simulink model "afe_abc_inv_psm_2mods"  (R2024b)
settings: Solver=ode1be  StartTime=0.0  StopTime=simlength  FixedStep=tc  MaxStep=tc
undefined symbols (not defined in the file): Adrso, afe_pwm_phase_shift_mod1, afe_pwm_phase_shift_mod2, Amplitude_U, Amplitude_V, Amplitude_W, Aresd, b, Bresd, Cresd, Crso, CTRPIFF_CLIP_RELEASE, dead_time_AFE, dead_time_INV, deepNEGeta, deepNEGxi, deepPOSxi, emf_fb_p, emf_fb_p_ccaller_1, emf_fb_p_ccaller_2, emf_p, emf_p_ccaller_1, emf_p_ccaller_2, enable_two_modules, end_time_LVRT, fPWM_AFE, fPWM_INV, g0_161Hz, g0_500Hz, g1_161Hz, g1_500Hz, i_grid_neg_eta_lim, i_grid_neg_eta_red_lim, i_grid_neg_xi_lim, i_grid_neg_xi_red_lim, i_grid_pos_eta_lim, i_grid_pos_eta_red_lim, ibez, id_lim, ieta_neg_ref_lim, ieta_pos_ref_lim, Igrid_phase_normalization_factor, inv_pwm_phase_shift_mod1, inv_pwm_phase_shift_mod2, iq_lim, ixi_pos_ref_lim, Jm, k_frt_ref, kg, ki_afe, ki_i, ki_rc_neg_grid, ki_rc_pos_grid, ki_vs, ki_w, kp_afe, kp_i, kp_rc_neg_grid, kp_rc_pos_grid, kp_vs ... (+59)
libraries: spsSampleandHoldLib x210, fl_lib x202, nesl_utility x126, simulink x22, cstblocks x18, threephase_inductor_lib x4, single_phase_transformer_lib x3, flexshaft_lib x1, pmsm_uvw_with_harmonics_lib x1
(part 6 of 18)

== system afe_abc_inv_psm_2mods/grid/grid_emulator/3ph_Dyg ==
  Electrical Reference1 : fl_lib/Electrical/Electrical Elements/Electrical Reference
  ph1 : single_phase_transformer_lib/single phase transformer  Lm=Lmu2_trafo H  n1=50*sqrt(3)  n2=50  Rd1=0 Ohm  Rd2=Rd2_trafo Ohm  Ld1=0 H  Ld2=Ld2_trafo H  Rfe=Rm2_trafo Ohm  phi_specify=off  phi_priority=None  phi=0 V*s  phi_nominal_specify=off  phi_nominal_value=1  phi_nominal_unit=V*s  i1_specify=off  i1_priority=None  i1=0 A  i1_nominal_specify=off  i1_nominal_value=1  i1_nominal_unit=A  i2_specify=off  i2_priority=None  i2=0 A  i2_nominal_specify=off  i2_nominal_value=1  i2_nominal_unit=A  ife_specify=off  ife_priority=None  ife=0 A  ife_nominal_specify=off  ife_nominal_value=1  ife_nominal_unit=A  u1_specify=off  u1_priority=None  u1=0 V  u1_nominal_specify=off  u1_nominal_value=1  u1_nominal_unit=V  u2_specify=off  u2_priority=None  u2=0 V  u2_nominal_specify=off  u2_nominal_value=1  u2_nominal_unit=V
      settings: InternalSimscapePortConfiguration="{\"Bottom\":[],\"Left\":[{\"id\":\"u1_p\",\"label\":\"u1(+)\",\"type\":\"foundation.electrical.electrical\"},{\"id\":\"u1_n\",\"label\":\"u1(-)\",\"type\":\"foundation.electrical.electrical\"}],\"Right\":[{\"id\":\"u2_p\",\"label\":\"u2(+)\",\"type\":\"foundation.electrical.electrical\"},{\"id\":\"u2_n\",\"label\":\"u2(-)\",\"type\":\"foundation.electrical.electrical\"}],\"Top\":[]}"
  ph2 : single_phase_transformer_lib/single phase transformer  Lm=Lmu2_trafo H  n1=50*sqrt(3)  n2=50  Rd1=0 Ohm  Rd2=Rd2_trafo Ohm  Ld1=0 H  Ld2=Ld2_trafo H  Rfe=Rm2_trafo Ohm  phi_specify=off  phi_priority=None  phi=0 V*s  phi_nominal_specify=off  phi_nominal_value=1  phi_nominal_unit=V*s  i1_specify=off  i1_priority=None  i1=0 A  i1_nominal_specify=off  i1_nominal_value=1  i1_nominal_unit=A  i2_specify=off  i2_priority=None  i2=0 A  i2_nominal_specify=off  i2_nominal_value=1  i2_nominal_unit=A  ife_specify=off  ife_priority=None  ife=0 A  ife_nominal_specify=off  ife_nominal_value=1  ife_nominal_unit=A  u1_specify=off  u1_priority=None  u1=0 V  u1_nominal_specify=off  u1_nominal_value=1  u1_nominal_unit=V  u2_specify=off  u2_priority=None  u2=0 V  u2_nominal_specify=off  u2_nominal_value=1  u2_nominal_unit=V
      settings: InternalSimscapePortConfiguration="{\"Bottom\":[],\"Left\":[{\"id\":\"u1_p\",\"label\":\"u1(+)\",\"type\":\"foundation.electrical.electrical\"},{\"id\":\"u1_n\",\"label\":\"u1(-)\",\"type\":\"foundation.electrical.electrical\"}],\"Right\":[{\"id\":\"u2_p\",\"label\":\"u2(+)\",\"type\":\"foundation.electrical.electrical\"},{\"id\":\"u2_n\",\"label\":\"u2(-)\",\"type\":\"foundation.electrical.electrical\"}],\"Top\":[]}"
  ph3 : single_phase_transformer_lib/single phase transformer  Lm=Lmu2_trafo H  n1=50*sqrt(3)  n2=50  Rd1=0 Ohm  Rd2=Rd2_trafo Ohm  Ld1=0 H  Ld2=Ld2_trafo H  Rfe=Rm2_trafo Ohm  phi_specify=off  phi_priority=None  phi=0 V*s  phi_nominal_specify=off  phi_nominal_value=1  phi_nominal_unit=V*s  i1_specify=off  i1_priority=None  i1=0 A  i1_nominal_specify=off  i1_nominal_value=1  i1_nominal_unit=A  i2_specify=off  i2_priority=None  i2=0 A  i2_nominal_specify=off  i2_nominal_value=1  i2_nominal_unit=A  ife_specify=off  ife_priority=None  ife=0 A  ife_nominal_specify=off  ife_nominal_value=1  ife_nominal_unit=A  u1_specify=off  u1_priority=None  u1=0 V  u1_nominal_specify=off  u1_nominal_value=1  u1_nominal_unit=V  u2_specify=off  u2_priority=None  u2=0 V  u2_nominal_specify=off  u2_nominal_value=1  u2_nominal_unit=V
      settings: InternalSimscapePortConfiguration="{\"Bottom\":[],\"Left\":[{\"id\":\"u1_p\",\"label\":\"u1(+)\",\"type\":\"foundation.electrical.electrical\"},{\"id\":\"u1_n\",\"label\":\"u1(-)\",\"type\":\"foundation.electrical.electrical\"}],\"Right\":[{\"id\":\"u2_p\",\"label\":\"u2(+)\",\"type\":\"foundation.electrical.electrical\"},{\"id\":\"u2_n\",\"label\":\"u2(-)\",\"type\":\"foundation.electrical.electrical\"}],\"Top\":[]}"
  ua : PMIOPort  Side=Right
  ub : PMIOPort  Port=2  Side=Right
  uc : PMIOPort  Port=3  Side=Right
  Ua : PMIOPort  Port=4  Side=Left
  Ub : PMIOPort  Port=5  Side=Left
  Uc : PMIOPort  Port=6  Side=Left
  connections:
  Electrical Reference1/LConn1 -- ph3/RConn2 -- ph2/RConn2 -- ph1/RConn2
  ph3/RConn1 -- uc/RConn1
  ph1/LConn1 -- ph3/LConn2 -- Ua/RConn1
  ph1/RConn1 -- ua/RConn1
  ph2/RConn1 -- ub/RConn1
  ph1/LConn2 -- ph2/LConn1 -- Ub/RConn1
  Uc/RConn1 -- ph3/LConn1 -- ph2/LConn2

== system afe_abc_inv_psm_2mods/grid/grid_emulator/grid_emulator ==
  phase_gen : Subsystem
  voltage_reference : Subsystem
  voltage_source : Subsystem
  Vma : Outport
  Vmb : Outport  Port=2
  Vmc : Outport  Port=3
  wires:
  phase_gen/1(grid_emu_phase) -> voltage_reference/1(grid_emu_phase)  "grid_emu_phase"
  voltage_source/2(vn_xi) -> voltage_reference/3(Vxi_n)
  voltage_source/1(vp_xi) -> voltage_reference/2(Vxi_p)
  voltage_source/3(vn_eta) -> voltage_reference/4(Veta_n)
  voltage_reference/3(V3_ref) -> Vmc/1
  voltage_reference/1(V1_ref) -> Vma/1
  voltage_reference/2(V2_ref) -> Vmb/1

== system afe_abc_inv_psm_2mods/grid/grid_emulator/threephase_vi_measures ==
  Bus Creator : BusCreator  Inputs=6
  Current Sensor : fl_lib/Electrical/Electrical Sensors/Current Sensor
  Current Sensor1 : fl_lib/Electrical/Electrical Sensors/Current Sensor
  Current Sensor2 : fl_lib/Electrical/Electrical Sensors/Current Sensor
  Electrical Reference1 : fl_lib/Electrical/Electrical Elements/Electrical Reference
  Voltage Sensor : fl_lib/Electrical/Electrical Sensors/Voltage Sensor
  Voltage Sensor1 : fl_lib/Electrical/Electrical Sensors/Voltage Sensor
  Voltage Sensor2 : fl_lib/Electrical/Electrical Sensors/Voltage Sensor
  i : Selector  InputPortWidth=6  IndexOptions=Index vector (dialog)  Indices=[4 5 6]  OutputSizes=1
  i_line_abc/u_line_abc : Scope  NumInputPorts=2
  ia_grid : nesl_utility/PS-Simulink Converter  PhysicalDomain=network_engine_domain  SubClassName=ps_output  LeftPortType=input  RightPortType=output  PseudoPeriodic=off  Frequencies=[]  VectorFormat=1-D array  Unit=A  AffineConversion=off
  ib_grid : nesl_utility/PS-Simulink Converter  PhysicalDomain=network_engine_domain  SubClassName=ps_output  LeftPortType=input  RightPortType=output  PseudoPeriodic=off  Frequencies=[]  VectorFormat=1-D array  Unit=A  AffineConversion=off
  ic_grid : nesl_utility/PS-Simulink Converter  PhysicalDomain=network_engine_domain  SubClassName=ps_output  LeftPortType=input  RightPortType=output  PseudoPeriodic=off  Frequencies=[]  VectorFormat=1-D array  Unit=A  AffineConversion=off
  u : Selector  InputPortWidth=6  IndexOptions=Index vector (dialog)  Indices=[1 2 3]  OutputSizes=1
  ua_grid : nesl_utility/PS-Simulink Converter  PhysicalDomain=network_engine_domain  SubClassName=ps_output  LeftPortType=input  RightPortType=output  PseudoPeriodic=off  Frequencies=[]  VectorFormat=1-D array  Unit=V  AffineConversion=off
  ub_grid : nesl_utility/PS-Simulink Converter  PhysicalDomain=network_engine_domain  SubClassName=ps_output  LeftPortType=input  RightPortType=output  PseudoPeriodic=off  Frequencies=[]  VectorFormat=1-D array  Unit=V  AffineConversion=off
  uc_grid : nesl_utility/PS-Simulink Converter  PhysicalDomain=network_engine_domain  SubClassName=ps_output  LeftPortType=input  RightPortType=output  PseudoPeriodic=off  Frequencies=[]  VectorFormat=1-D array  Unit=V  AffineConversion=off
  Ua : PMIOPort  Side=Left
  ua : PMIOPort  Port=2  Side=Right
  Ub : PMIOPort  Port=3  Side=Left
  ub : PMIOPort  Port=4  Side=Right
  Uc : PMIOPort  Port=5  Side=Left
  uc : PMIOPort  Port=6  Side=Right
  wires:
  Bus Creator/1 -> i/1, u/1  "vi_data"
  ib_grid/1 -> Bus Creator/5  "ib"
  ia_grid/1 -> Bus Creator/4  "ia"
  ic_grid/1 -> Bus Creator/6  "ic"
  ua_grid/1 -> Bus Creator/1  "ua"
  ub_grid/1 -> Bus Creator/2  "ub"
  uc_grid/1 -> Bus Creator/3  "uc"
  i/1 -> i_line_abc/u_line_abc/1
  u/1 -> i_line_abc/u_line_abc/2
  connections:
  Current Sensor1/LConn1 -- Ub/RConn1 -- Voltage Sensor1/LConn1
  Electrical Reference1/LConn1 -- Voltage Sensor/RConn2 -- Voltage Sensor2/RConn2 -- Voltage Sensor1/RConn2
  Voltage Sensor/RConn1 -- ua_grid/LConn1
  Current Sensor/RConn2 -- ua/RConn1
  Voltage Sensor1/RConn1 -- ub_grid/LConn1
  Voltage Sensor2/LConn1 -- Current Sensor2/LConn1 -- Uc/RConn1
  Current Sensor/LConn1 -- Ua/RConn1 -- Voltage Sensor/LConn1
  Current Sensor1/RConn2 -- ub/RConn1
  Voltage Sensor2/RConn1 -- uc_grid/LConn1
  ib_grid/LConn1 -- Current Sensor1/RConn1
  ia_grid/LConn1 -- Current Sensor/RConn1
  ic_grid/LConn1 -- Current Sensor2/RConn1
  Current Sensor2/RConn2 -- uc/RConn1

== system afe_abc_inv_psm_2mods/grid/instantaneus_power/abc2alphabeta ==
  a : Inport
  b : Inport  Port=2
  c : Inport  Port=3
  Gain1 : Gain  Gain=-1/2
  Gain11 : Gain  Gain=-1/2
  Gain2 : Gain  Gain=0
  Gain3 : Gain  Gain=sqrt(3)/2
  Gain4 : Gain  Gain=-sqrt(3)/2
  Gain8 : Gain  Gain=2/3
  Gain9 : Gain  Gain=2/3
  Sum : Sum  Inputs=+++
  Sum1 : Sum  Inputs=+++
  "alpha " : Outport  VectorParamsAs1DForOutWhenUnconnected=off
  "beta " : Outport  Port=2  VectorParamsAs1DForOutWhenUnconnected=off
  wires:
  Gain3/1 -> Sum1/2
  Gain2/1 -> Sum1/1
  Gain11/1 -> Sum/2
  Gain4/1 -> Sum1/3
  Sum1/1 -> Gain9/1
  Gain8/1 -> "alpha "/1
  Sum/1 -> Gain8/1
  c/1 -> Gain4/1, Gain1/1
  Gain9/1 -> "beta "/1
  b/1 -> Gain3/1, Gain11/1
  Gain1/1 -> Sum/3
  a/1 -> Gain2/1, Sum/1

== system afe_abc_inv_psm_2mods/grid/instantaneus_power/abc2alphabeta  ==
  a : Inport
  b : Inport  Port=2
  c : Inport  Port=3
  Gain1 : Gain  Gain=-1/2
  Gain11 : Gain  Gain=-1/2
  Gain2 : Gain  Gain=0
  Gain3 : Gain  Gain=sqrt(3)/2
  Gain4 : Gain  Gain=-sqrt(3)/2
  Gain8 : Gain  Gain=2/3
  Gain9 : Gain  Gain=2/3
  Sum : Sum  Inputs=+++
  Sum1 : Sum  Inputs=+++
  "alpha " : Outport  VectorParamsAs1DForOutWhenUnconnected=off
  "beta " : Outport  Port=2  VectorParamsAs1DForOutWhenUnconnected=off
  wires:
  a/1 -> Sum/1, Gain2/1
  Gain2/1 -> Sum1/1
  Gain9/1 -> "beta "/1
  Gain11/1 -> Sum/2
  c/1 -> Gain1/1, Gain4/1
  Sum/1 -> Gain8/1
  Sum1/1 -> Gain9/1
  Gain1/1 -> Sum/3
  Gain3/1 -> Sum1/2
  Gain4/1 -> Sum1/3
  Gain8/1 -> "alpha "/1
  b/1 -> Gain11/1, Gain3/1

== system afe_abc_inv_psm_2mods/grid/instantaneus_power/moving_avarage ==
  In : Inport
  Gain1 : Gain  Gain=omega_grid_emulator_nom/2/pi  SaturateOnIntegerOverflow=on  OutDataTypeStr=Inherit: Same as input  ParamDataTypeStr=Inherit: Same as input
  Sum4 : Sum  SaturateOnIntegerOverflow=on
  Sum8 : Sum  Inputs=+-  InputSameDT=on  SaturateOnIntegerOverflow=on  OutDataTypeStr=Inherit: Same as first input
  Transport Delay : TransportDelay  DelayTime=2*pi/omega_grid_emulator_nom  BufferSize=2048*4  PadeOrder=2
  Unit Delay2 : UnitDelay  SampleTime=ts_afe  HasFrameUpgradeWarning=on
  kp2 : Gain  Gain=ts_afe  SaturateOnIntegerOverflow=on  OutDataTypeStr=Inherit: Same as input  ParamDataTypeStr=Inherit: Same as input
  Mean : Outport  VectorParamsAs1DForOutWhenUnconnected=off
  wires:
  Transport Delay/1 -> Sum8/2
  Sum4/1 -> Sum8/1, Transport Delay/1, Unit Delay2/1
  Sum8/1 -> Gain1/1
  In/1 -> kp2/1
  Unit Delay2/1 -> Sum4/2
  kp2/1 -> Sum4/1
  Gain1/1 -> Mean/1

== system afe_abc_inv_psm_2mods/grid/instantaneus_power/moving_avarage1 ==
  In : Inport
  Gain1 : Gain  Gain=omega_grid_emulator_nom/2/pi  SaturateOnIntegerOverflow=on  OutDataTypeStr=Inherit: Same as input  ParamDataTypeStr=Inherit: Same as input
  Sum4 : Sum  SaturateOnIntegerOverflow=on
  Sum8 : Sum  Inputs=+-  InputSameDT=on  SaturateOnIntegerOverflow=on  OutDataTypeStr=Inherit: Same as first input
  Transport Delay : TransportDelay  DelayTime=2*pi/omega_grid_emulator_nom  BufferSize=2048*4  PadeOrder=2
  Unit Delay2 : UnitDelay  SampleTime=ts_afe  HasFrameUpgradeWarning=on
  kp2 : Gain  Gain=ts_afe  SaturateOnIntegerOverflow=on  OutDataTypeStr=Inherit: Same as input  ParamDataTypeStr=Inherit: Same as input
  Mean : Outport  VectorParamsAs1DForOutWhenUnconnected=off
  wires:
  Gain1/1 -> Mean/1
  kp2/1 -> Sum4/1
  Unit Delay2/1 -> Sum4/2
  In/1 -> kp2/1
  Sum8/1 -> Gain1/1
  Sum4/1 -> Unit Delay2/1, Transport Delay/1, Sum8/1
  Transport Delay/1 -> Sum8/2

== system afe_abc_inv_psm_2mods/grid/instantaneus_power/rms ==
  In1 : Inport
  Gain : Gain  Gain=n10-1
  Gain1 : Gain  Gain=1/n10
  Math Function : Math  Operator=magnitude^2  SignedPower=on
  Sqrt : Sqrt
  Sum : Sum  Inputs=|++
  Unit Delay : UnitDelay  SampleTime=ts_afe  HasFrameUpgradeWarning=on
  Out1 : Outport  VectorParamsAs1DForOutWhenUnconnected=off
  wires:
  In1/1 -> Math Function/1
  Sum/1 -> Gain1/1
  Gain1/1 -> Sqrt/1, Unit Delay/1
  Unit Delay/1 -> Gain/1
  Math Function/1 -> Sum/1
  Sqrt/1 -> Out1/1
  Gain/1 -> Sum/2

== system afe_abc_inv_psm_2mods/grid/instantaneus_power/rms1 ==
  In1 : Inport
  Gain : Gain  Gain=n10-1
  Gain1 : Gain  Gain=1/n10
  Math Function : Math  Operator=magnitude^2  SignedPower=on
  Sqrt : Sqrt
  Sum : Sum  Inputs=|++
  Unit Delay : UnitDelay  SampleTime=ts_afe  HasFrameUpgradeWarning=on
  Out1 : Outport  VectorParamsAs1DForOutWhenUnconnected=off
  wires:
  Gain/1 -> Sum/2
  Sqrt/1 -> Out1/1
  Math Function/1 -> Sum/1
  Unit Delay/1 -> Gain/1
  Gain1/1 -> Unit Delay/1, Sqrt/1
  Sum/1 -> Gain1/1
  In1/1 -> Math Function/1

== system afe_abc_inv_psm_2mods/grid/instantaneus_power/rms2 ==
  In1 : Inport
  Gain : Gain  Gain=n10-1
  Gain1 : Gain  Gain=1/n10
  Math Function : Math  Operator=magnitude^2  SignedPower=on
  Sqrt : Sqrt
  Sum : Sum  Inputs=|++
  Unit Delay : UnitDelay  SampleTime=ts_afe  HasFrameUpgradeWarning=on
  Out1 : Outport  VectorParamsAs1DForOutWhenUnconnected=off
  wires:
  In1/1 -> Math Function/1
  Sum/1 -> Gain1/1
  Gain1/1 -> Sqrt/1, Unit Delay/1
  Unit Delay/1 -> Gain/1
  Math Function/1 -> Sum/1
  Sqrt/1 -> Out1/1
  Gain/1 -> Sum/2

== system afe_abc_inv_psm_2mods/grid/instantaneus_power/rms3 ==
  In1 : Inport
  Gain : Gain  Gain=n10-1
  Gain1 : Gain  Gain=1/n10
  Math Function : Math  Operator=magnitude^2  SignedPower=on
  Sqrt : Sqrt
  Sum : Sum  Inputs=|++
  Unit Delay : UnitDelay  SampleTime=ts_afe  HasFrameUpgradeWarning=on
  Out1 : Outport  VectorParamsAs1DForOutWhenUnconnected=off
  wires:
  Gain/1 -> Sum/2
  Sqrt/1 -> Out1/1
  Math Function/1 -> Sum/1
  Unit Delay/1 -> Gain/1
  Gain1/1 -> Unit Delay/1, Sqrt/1
  Sum/1 -> Gain1/1
  In1/1 -> Math Function/1

== system afe_abc_inv_psm_2mods/grid/instantaneus_power/rms4 ==
  In1 : Inport
  Gain : Gain  Gain=n10-1
  Gain1 : Gain  Gain=1/n10
  Math Function : Math  Operator=magnitude^2  SignedPower=on
  Sqrt : Sqrt
  Sum : Sum  Inputs=|++
  Unit Delay : UnitDelay  SampleTime=ts_afe  HasFrameUpgradeWarning=on
  Out1 : Outport  VectorParamsAs1DForOutWhenUnconnected=off
  wires:
  In1/1 -> Math Function/1
  Sum/1 -> Gain1/1
  Gain1/1 -> Sqrt/1, Unit Delay/1
  Unit Delay/1 -> Gain/1
  Math Function/1 -> Sum/1
  Sqrt/1 -> Out1/1
  Gain/1 -> Sum/2

== system afe_abc_inv_psm_2mods/grid/instantaneus_power/rms5 ==
  In1 : Inport
  Gain : Gain  Gain=n10-1
  Gain1 : Gain  Gain=1/n10
  Math Function : Math  Operator=magnitude^2  SignedPower=on
  Sqrt : Sqrt
  Sum : Sum  Inputs=|++
  Unit Delay : UnitDelay  SampleTime=ts_afe  HasFrameUpgradeWarning=on
  Out1 : Outport  VectorParamsAs1DForOutWhenUnconnected=off
  wires:
  Gain/1 -> Sum/2
  Sqrt/1 -> Out1/1
  Math Function/1 -> Sum/1
  Unit Delay/1 -> Gain/1
  Gain1/1 -> Unit Delay/1, Sqrt/1
  Sum/1 -> Gain1/1
  In1/1 -> Math Function/1

== system afe_abc_inv_psm_2mods/grid/sequences/moving_avarage ==
  In : Inport
  Gain1 : Gain  Gain=omega_grid_emulator_nom/2/pi  SaturateOnIntegerOverflow=on  OutDataTypeStr=Inherit: Same as input  ParamDataTypeStr=Inherit: Same as input
  Sum4 : Sum  SaturateOnIntegerOverflow=on
  Sum8 : Sum  Inputs=+-  InputSameDT=on  SaturateOnIntegerOverflow=on  OutDataTypeStr=Inherit: Same as first input
  Transport Delay : TransportDelay  DelayTime=2*pi/omega_grid_emulator_nom  BufferSize=2048*4  PadeOrder=2
  Unit Delay2 : UnitDelay  SampleTime=ts_afe  HasFrameUpgradeWarning=on
  kp2 : Gain  Gain=ts_afe  SaturateOnIntegerOverflow=on  OutDataTypeStr=Inherit: Same as input  ParamDataTypeStr=Inherit: Same as input
  Mean : Outport  VectorParamsAs1DForOutWhenUnconnected=off
  wires:
  Transport Delay/1 -> Sum8/2
  Sum4/1 -> Sum8/1, Transport Delay/1, Unit Delay2/1
  Sum8/1 -> Gain1/1
  In/1 -> kp2/1
  Unit Delay2/1 -> Sum4/2
  kp2/1 -> Sum4/1
  Gain1/1 -> Mean/1

== system afe_abc_inv_psm_2mods/grid/sequences/moving_avarage1 ==
  In : Inport
  Gain1 : Gain  Gain=omega_grid_emulator_nom/2/pi  SaturateOnIntegerOverflow=on  OutDataTypeStr=Inherit: Same as input  ParamDataTypeStr=Inherit: Same as input
  Sum4 : Sum  SaturateOnIntegerOverflow=on
  Sum8 : Sum  Inputs=+-  InputSameDT=on  SaturateOnIntegerOverflow=on  OutDataTypeStr=Inherit: Same as first input
  Transport Delay : TransportDelay  DelayTime=2*pi/omega_grid_emulator_nom  BufferSize=2048*4  PadeOrder=2
  Unit Delay2 : UnitDelay  SampleTime=ts_afe  HasFrameUpgradeWarning=on
  kp2 : Gain  Gain=ts_afe  SaturateOnIntegerOverflow=on  OutDataTypeStr=Inherit: Same as input  ParamDataTypeStr=Inherit: Same as input
  Mean : Outport  VectorParamsAs1DForOutWhenUnconnected=off
  wires:
  Gain1/1 -> Mean/1
  kp2/1 -> Sum4/1
  Unit Delay2/1 -> Sum4/2
  In/1 -> kp2/1
  Sum8/1 -> Gain1/1
  Sum4/1 -> Unit Delay2/1, Transport Delay/1, Sum8/1
  Transport Delay/1 -> Sum8/2

== system afe_abc_inv_psm_2mods/grid/sequences/moving_avarage10 ==
  In : Inport
  Gain1 : Gain  Gain=omega_grid_emulator_nom/2/pi  SaturateOnIntegerOverflow=on  OutDataTypeStr=Inherit: Same as input  ParamDataTypeStr=Inherit: Same as input
  Sum4 : Sum  SaturateOnIntegerOverflow=on
  Sum8 : Sum  Inputs=+-  InputSameDT=on  SaturateOnIntegerOverflow=on  OutDataTypeStr=Inherit: Same as first input
  Transport Delay : TransportDelay  DelayTime=2*pi/omega_grid_emulator_nom  BufferSize=2048*4  PadeOrder=2
  Unit Delay2 : UnitDelay  SampleTime=ts_afe  HasFrameUpgradeWarning=on
  kp2 : Gain  Gain=ts_afe  SaturateOnIntegerOverflow=on  OutDataTypeStr=Inherit: Same as input  ParamDataTypeStr=Inherit: Same as input
  Mean : Outport  VectorParamsAs1DForOutWhenUnconnected=off
  wires:
  Transport Delay/1 -> Sum8/2
  Sum4/1 -> Sum8/1, Transport Delay/1, Unit Delay2/1
  Sum8/1 -> Gain1/1
  In/1 -> kp2/1
  Unit Delay2/1 -> Sum4/2
  kp2/1 -> Sum4/1
  Gain1/1 -> Mean/1

== system afe_abc_inv_psm_2mods/grid/sequences/moving_avarage11 ==
  In : Inport
  Gain1 : Gain  Gain=omega_grid_emulator_nom/2/pi  SaturateOnIntegerOverflow=on  OutDataTypeStr=Inherit: Same as input  ParamDataTypeStr=Inherit: Same as input
  Sum4 : Sum  SaturateOnIntegerOverflow=on
  Sum8 : Sum  Inputs=+-  InputSameDT=on  SaturateOnIntegerOverflow=on  OutDataTypeStr=Inherit: Same as first input
  Transport Delay : TransportDelay  DelayTime=2*pi/omega_grid_emulator_nom  BufferSize=2048*4  PadeOrder=2
  Unit Delay2 : UnitDelay  SampleTime=ts_afe  HasFrameUpgradeWarning=on
  kp2 : Gain  Gain=ts_afe  SaturateOnIntegerOverflow=on  OutDataTypeStr=Inherit: Same as input  ParamDataTypeStr=Inherit: Same as input
  Mean : Outport  VectorParamsAs1DForOutWhenUnconnected=off
  wires:
  Gain1/1 -> Mean/1
  kp2/1 -> Sum4/1
  Unit Delay2/1 -> Sum4/2
  In/1 -> kp2/1
  Sum8/1 -> Gain1/1
  Sum4/1 -> Unit Delay2/1, Transport Delay/1, Sum8/1
  Transport Delay/1 -> Sum8/2

== system afe_abc_inv_psm_2mods/grid/sequences/moving_avarage2 ==
  In : Inport
  Gain1 : Gain  Gain=omega_grid_emulator_nom/2/pi  SaturateOnIntegerOverflow=on  OutDataTypeStr=Inherit: Same as input  ParamDataTypeStr=Inherit: Same as input
  Sum4 : Sum  SaturateOnIntegerOverflow=on
  Sum8 : Sum  Inputs=+-  InputSameDT=on  SaturateOnIntegerOverflow=on  OutDataTypeStr=Inherit: Same as first input
  Transport Delay : TransportDelay  DelayTime=2*pi/omega_grid_emulator_nom  BufferSize=2048*4  PadeOrder=2
  Unit Delay2 : UnitDelay  SampleTime=ts_afe  HasFrameUpgradeWarning=on
  kp2 : Gain  Gain=ts_afe  SaturateOnIntegerOverflow=on  OutDataTypeStr=Inherit: Same as input  ParamDataTypeStr=Inherit: Same as input
  Mean : Outport  VectorParamsAs1DForOutWhenUnconnected=off
  wires:
  Transport Delay/1 -> Sum8/2
  Sum4/1 -> Sum8/1, Transport Delay/1, Unit Delay2/1
  Sum8/1 -> Gain1/1
  In/1 -> kp2/1
  Unit Delay2/1 -> Sum4/2
  kp2/1 -> Sum4/1
  Gain1/1 -> Mean/1

== system afe_abc_inv_psm_2mods/grid/sequences/moving_avarage3 ==
  In : Inport
  Gain1 : Gain  Gain=omega_grid_emulator_nom/2/pi  SaturateOnIntegerOverflow=on  OutDataTypeStr=Inherit: Same as input  ParamDataTypeStr=Inherit: Same as input
  Sum4 : Sum  SaturateOnIntegerOverflow=on
  Sum8 : Sum  Inputs=+-  InputSameDT=on  SaturateOnIntegerOverflow=on  OutDataTypeStr=Inherit: Same as first input
  Transport Delay : TransportDelay  DelayTime=2*pi/omega_grid_emulator_nom  BufferSize=2048*4  PadeOrder=2
  Unit Delay2 : UnitDelay  SampleTime=ts_afe  HasFrameUpgradeWarning=on
  kp2 : Gain  Gain=ts_afe  SaturateOnIntegerOverflow=on  OutDataTypeStr=Inherit: Same as input  ParamDataTypeStr=Inherit: Same as input
  Mean : Outport  VectorParamsAs1DForOutWhenUnconnected=off
  wires:
  Gain1/1 -> Mean/1
  kp2/1 -> Sum4/1
  Unit Delay2/1 -> Sum4/2
  In/1 -> kp2/1
  Sum8/1 -> Gain1/1
  Sum4/1 -> Unit Delay2/1, Transport Delay/1, Sum8/1
  Transport Delay/1 -> Sum8/2

== system afe_abc_inv_psm_2mods/grid/sequences/moving_avarage4 ==
  In : Inport
  Gain1 : Gain  Gain=omega_grid_emulator_nom/2/pi  SaturateOnIntegerOverflow=on  OutDataTypeStr=Inherit: Same as input  ParamDataTypeStr=Inherit: Same as input
  Sum4 : Sum  SaturateOnIntegerOverflow=on
  Sum8 : Sum  Inputs=+-  InputSameDT=on  SaturateOnIntegerOverflow=on  OutDataTypeStr=Inherit: Same as first input
  Transport Delay : TransportDelay  DelayTime=2*pi/omega_grid_emulator_nom  BufferSize=2048*4  PadeOrder=2
  Unit Delay2 : UnitDelay  SampleTime=ts_afe  HasFrameUpgradeWarning=on
  kp2 : Gain  Gain=ts_afe  SaturateOnIntegerOverflow=on  OutDataTypeStr=Inherit: Same as input  ParamDataTypeStr=Inherit: Same as input
  Mean : Outport  VectorParamsAs1DForOutWhenUnconnected=off
  wires:
  Transport Delay/1 -> Sum8/2
  Sum4/1 -> Sum8/1, Transport Delay/1, Unit Delay2/1
  Sum8/1 -> Gain1/1
  In/1 -> kp2/1
  Unit Delay2/1 -> Sum4/2
  kp2/1 -> Sum4/1
  Gain1/1 -> Mean/1

== system afe_abc_inv_psm_2mods/grid/sequences/moving_avarage5 ==
  In : Inport
  Gain1 : Gain  Gain=omega_grid_emulator_nom/2/pi  SaturateOnIntegerOverflow=on  OutDataTypeStr=Inherit: Same as input  ParamDataTypeStr=Inherit: Same as input
  Sum4 : Sum  SaturateOnIntegerOverflow=on
  Sum8 : Sum  Inputs=+-  InputSameDT=on  SaturateOnIntegerOverflow=on  OutDataTypeStr=Inherit: Same as first input
  Transport Delay : TransportDelay  DelayTime=2*pi/omega_grid_emulator_nom  BufferSize=2048*4  PadeOrder=2
  Unit Delay2 : UnitDelay  SampleTime=ts_afe  HasFrameUpgradeWarning=on
  kp2 : Gain  Gain=ts_afe  SaturateOnIntegerOverflow=on  OutDataTypeStr=Inherit: Same as input  ParamDataTypeStr=Inherit: Same as input
  Mean : Outport  VectorParamsAs1DForOutWhenUnconnected=off
  wires:
  Gain1/1 -> Mean/1
  kp2/1 -> Sum4/1
  Unit Delay2/1 -> Sum4/2
  In/1 -> kp2/1
  Sum8/1 -> Gain1/1
  Sum4/1 -> Unit Delay2/1, Transport Delay/1, Sum8/1
  Transport Delay/1 -> Sum8/2

== system afe_abc_inv_psm_2mods/grid/sequences/moving_avarage6 ==
  In : Inport
  Gain1 : Gain  Gain=omega_grid_emulator_nom/2/pi  SaturateOnIntegerOverflow=on  OutDataTypeStr=Inherit: Same as input  ParamDataTypeStr=Inherit: Same as input
  Sum4 : Sum  SaturateOnIntegerOverflow=on
  Sum8 : Sum  Inputs=+-  InputSameDT=on  SaturateOnIntegerOverflow=on  OutDataTypeStr=Inherit: Same as first input
  Transport Delay : TransportDelay  DelayTime=2*pi/omega_grid_emulator_nom  BufferSize=2048*4  PadeOrder=2
  Unit Delay2 : UnitDelay  SampleTime=ts_afe  HasFrameUpgradeWarning=on
  kp2 : Gain  Gain=ts_afe  SaturateOnIntegerOverflow=on  OutDataTypeStr=Inherit: Same as input  ParamDataTypeStr=Inherit: Same as input
  Mean : Outport  VectorParamsAs1DForOutWhenUnconnected=off
  wires:
  Transport Delay/1 -> Sum8/2
  Sum4/1 -> Sum8/1, Transport Delay/1, Unit Delay2/1
  Sum8/1 -> Gain1/1
  In/1 -> kp2/1
  Unit Delay2/1 -> Sum4/2
  kp2/1 -> Sum4/1
  Gain1/1 -> Mean/1

== system afe_abc_inv_psm_2mods/grid/sequences/moving_avarage7 ==
  In : Inport
  Gain1 : Gain  Gain=omega_grid_emulator_nom/2/pi  SaturateOnIntegerOverflow=on  OutDataTypeStr=Inherit: Same as input  ParamDataTypeStr=Inherit: Same as input
  Sum4 : Sum  SaturateOnIntegerOverflow=on
  Sum8 : Sum  Inputs=+-  InputSameDT=on  SaturateOnIntegerOverflow=on  OutDataTypeStr=Inherit: Same as first input
  Transport Delay : TransportDelay  DelayTime=2*pi/omega_grid_emulator_nom  BufferSize=2048*4  PadeOrder=2
  Unit Delay2 : UnitDelay  SampleTime=ts_afe  HasFrameUpgradeWarning=on
  kp2 : Gain  Gain=ts_afe  SaturateOnIntegerOverflow=on  OutDataTypeStr=Inherit: Same as input  ParamDataTypeStr=Inherit: Same as input
  Mean : Outport  VectorParamsAs1DForOutWhenUnconnected=off
  wires:
  Gain1/1 -> Mean/1
  kp2/1 -> Sum4/1
  Unit Delay2/1 -> Sum4/2
  In/1 -> kp2/1
  Sum8/1 -> Gain1/1
  Sum4/1 -> Unit Delay2/1, Transport Delay/1, Sum8/1
  Transport Delay/1 -> Sum8/2

== system afe_abc_inv_psm_2mods/grid/sequences/moving_avarage8 ==
  In : Inport
  Gain1 : Gain  Gain=omega_grid_emulator_nom/2/pi  SaturateOnIntegerOverflow=on  OutDataTypeStr=Inherit: Same as input  ParamDataTypeStr=Inherit: Same as input
  Sum4 : Sum  SaturateOnIntegerOverflow=on
  Sum8 : Sum  Inputs=+-  InputSameDT=on  SaturateOnIntegerOverflow=on  OutDataTypeStr=Inherit: Same as first input
  Transport Delay : TransportDelay  DelayTime=2*pi/omega_grid_emulator_nom  BufferSize=2048*4  PadeOrder=2
  Unit Delay2 : UnitDelay  SampleTime=ts_afe  HasFrameUpgradeWarning=on
  kp2 : Gain  Gain=ts_afe  SaturateOnIntegerOverflow=on  OutDataTypeStr=Inherit: Same as input  ParamDataTypeStr=Inherit: Same as input
  Mean : Outport  VectorParamsAs1DForOutWhenUnconnected=off
  wires:
  Transport Delay/1 -> Sum8/2
  Sum4/1 -> Sum8/1, Transport Delay/1, Unit Delay2/1
  Sum8/1 -> Gain1/1
  In/1 -> kp2/1
  Unit Delay2/1 -> Sum4/2
  kp2/1 -> Sum4/1
  Gain1/1 -> Mean/1

== system afe_abc_inv_psm_2mods/grid/sequences/moving_avarage9 ==
  In : Inport
  Gain1 : Gain  Gain=omega_grid_emulator_nom/2/pi  SaturateOnIntegerOverflow=on  OutDataTypeStr=Inherit: Same as input  ParamDataTypeStr=Inherit: Same as input
  Sum4 : Sum  SaturateOnIntegerOverflow=on
  Sum8 : Sum  Inputs=+-  InputSameDT=on  SaturateOnIntegerOverflow=on  OutDataTypeStr=Inherit: Same as first input
  Transport Delay : TransportDelay  DelayTime=2*pi/omega_grid_emulator_nom  BufferSize=2048*4  PadeOrder=2
  Unit Delay2 : UnitDelay  SampleTime=ts_afe  HasFrameUpgradeWarning=on
  kp2 : Gain  Gain=ts_afe  SaturateOnIntegerOverflow=on  OutDataTypeStr=Inherit: Same as input  ParamDataTypeStr=Inherit: Same as input
  Mean : Outport  VectorParamsAs1DForOutWhenUnconnected=off
  wires:
  Gain1/1 -> Mean/1
  kp2/1 -> Sum4/1
  Unit Delay2/1 -> Sum4/2
  In/1 -> kp2/1
  Sum8/1 -> Gain1/1
  Sum4/1 -> Unit Delay2/1, Transport Delay/1, Sum8/1
  Transport Delay/1 -> Sum8/2

== system afe_abc_inv_psm_2mods/afe_abc_inv_psm_mod1/afe/dclink_measure/R_derating ==
  Step : Step  After=107.4e3/2  SampleTime=0
  Step1 : Step  Time=1.1  After=-107.4e3/2  SampleTime=0
  Sum : Sum  Inputs=|++
  DR : Outport
  wires:
  Step1/1 -> Sum/2
  Step/1 -> Sum/1
  Sum/1 -> DR/1

== system afe_abc_inv_psm_2mods/afe_abc_inv_psm_mod1/afe/dclink_measure/Subsystem1 ==
  In : Inport
  Sample and Hold : spsSampleandHoldLib/Sample and Hold  ic=0  Ts=0
  Out : Outport
  wires:
  Sample and Hold/1 -> Out/1
  [TRGO_afe_module_1] -> Sample and Hold/2
  In/1 -> Sample and Hold/1

== system afe_abc_inv_psm_2mods/afe_abc_inv_psm_mod1/afe/dclink_measure/Subsystem2 ==
  In : Inport
  Sample and Hold : spsSampleandHoldLib/Sample and Hold  ic=0  Ts=0
  Out : Outport
  wires:
  Sample and Hold/1 -> Out/1
  [TRGO_inv_module_1] -> Sample and Hold/2
  In/1 -> Sample and Hold/1

== system afe_abc_inv_psm_2mods/afe_abc_inv_psm_mod1/afe/sv_pwm/Subsystem1 ==
  In : Inport
  Sample and Hold : spsSampleandHoldLib/Sample and Hold  ic=0  Ts=0
  Out : Outport
  wires:
  In/1 -> Sample and Hold/1
  [TRGO_afe_module_1] -> Sample and Hold/2
  Sample and Hold/1 -> Out/1

== system afe_abc_inv_psm_2mods/afe_abc_inv_psm_mod1/afe/sv_pwm/Subsystem2 ==
  In : Inport
  Sample and Hold : spsSampleandHoldLib/Sample and Hold  ic=0  Ts=0
  Out : Outport
  wires:
  Sample and Hold/1 -> Out/1
  [TRGO_afe_module_1] -> Sample and Hold/2
  In/1 -> Sample and Hold/1

== system afe_abc_inv_psm_2mods/afe_abc_inv_psm_mod1/afe/sv_pwm/Subsystem4 ==
  In : Inport
  Sample and Hold : spsSampleandHoldLib/Sample and Hold  ic=0  Ts=0
  Out : Outport
  wires:
  Sample and Hold/1 -> Out/1
  [TRGO_afe_module_1] -> Sample and Hold/2
  In/1 -> Sample and Hold/1

== system afe_abc_inv_psm_2mods/afe_abc_inv_psm_mod1/afe/sv_pwm/Subsystem5 ==
  In : Inport
  Sample and Hold : spsSampleandHoldLib/Sample and Hold  ic=0  Ts=0
  Out : Outport
  wires:
  In/1 -> Sample and Hold/1
  [TRGO_afe_module_1] -> Sample and Hold/2
  Sample and Hold/1 -> Out/1

== system afe_abc_inv_psm_2mods/afe_abc_inv_psm_mod1/afe/sv_pwm/modulator1 ==
  u : Inport
  v : Inport  Port=2
  w : Inport  Port=3
  phase : Inport  Port=4
  Bus Creator3 : BusCreator  Inputs=6
  PWM generator 1 : Subsystem  mask{f=fPWM_AFE, m_up=0.98, m_low=0.02, dead_time=dead_time_AFE, pos_cmd_gate=15, neg_cmd_gate=-10, polarity=1}
      mask prompts: f "Frequency (Hz)"; m_up "Max Input Modulation Value"; m_low "Min Input Modulation Value"; dead_time "Dead Time (s)"; pos_cmd_gate "Positive Gate Voltage (V)"; neg_cmd_gate "Negative Gate Voltage (V)"; polarity "Polarity (pu)"
  PWM generator 2 : Subsystem  mask{f=fPWM_AFE, m_up=0.98, m_low=0.02, dead_time=dead_time_AFE, pos_cmd_gate=15, neg_cmd_gate=-10, polarity=1}
      mask prompts: f "Frequency (Hz)"; m_up "Max Input Modulation Value"; m_low "Min Input Modulation Value"; dead_time "Dead Time (s)"; pos_cmd_gate "Positive Gate Voltage (V)"; neg_cmd_gate "Negative Gate Voltage (V)"; polarity "Polarity (pu)"
  PWM generator 3 : Subsystem  mask{f=fPWM_AFE, m_up=0.98, m_low=0.02, dead_time=dead_time_AFE, pos_cmd_gate=15, neg_cmd_gate=-10, polarity=1}
      mask prompts: f "Frequency (Hz)"; m_up "Max Input Modulation Value"; m_low "Min Input Modulation Value"; dead_time "Dead Time (s)"; pos_cmd_gate "Positive Gate Voltage (V)"; neg_cmd_gate "Negative Gate Voltage (V)"; polarity "Polarity (pu)"
  cmd_gates : Outport
  wires:
  u/1 -> PWM generator 1/1(m_index)
  w/1 -> PWM generator 3/1(m_index)
  v/1 -> PWM generator 2/1(m_index)
  phase/1 -> PWM generator 3/2(phase), PWM generator 2/2(phase), PWM generator 1/2(phase)
  PWM generator 1/2(m2) -> Bus Creator3/2  "pwm_afe_phase_u_bottom"
  PWM generator 3/1(m1) -> Bus Creator3/5  "pwm_afe_phase_w_top"
  PWM generator 2/1(m1) -> Bus Creator3/3  "pwm_afe_phase_v_top"
  PWM generator 2/2(m2) -> Bus Creator3/4  "pwm_afe_phase_v_bottom"
  PWM generator 3/2(m2) -> Bus Creator3/6  "pwm_afe_phase_w_bottom"
  PWM generator 1/1(m1) -> Bus Creator3/1  "pwm_afe_phase_u_top"
  Bus Creator3/1 -> cmd_gates/1

== system afe_abc_inv_psm_2mods/afe_abc_inv_psm_mod1/afe_control/FRT-VDE4110/FRT-Detection ==
  red_dyn_enabled : Inport
  Abs : Abs  SaturateOnIntegerOverflow=off
  Abs1 : Abs  SaturateOnIntegerOverflow=off
  LVRT_detector : MATLAB Function  TreatAsAtomicUnit=on  SystemSampleTime=ts_afe
  Step1 : Step  Time=0.025  Before=1  After=0  SampleTime=ts_afe
  Step3 : Step  Time=settle_time  SampleTime=ts_afe
  dvxi_n/dt : Subsystem
  dvxi_p/dt : Subsystem
  frt_detection_inputs : Scope  NumInputPorts=6
  frt_exceeded : Outport
  frt_state : Outport  Port=2
  red_dyn_active : Outport  Port=3
  frt_active : Outport  Port=4
  pwr_lim_enable : Outport  Port=5
  wires:
  [v_grid_neg_xi_avg_mod1] -> LVRT_detector/2(vxi_n), frt_detection_inputs/2, dvxi_n/dt/1(x)  "v_grid_neg_xi_avg"
  [v_grid_pos_xi_avg_mod1] -> LVRT_detector/1(vxi_p), frt_detection_inputs/1, dvxi_p/dt/1(x)  "v_grid_pos_xi_avg"
  [v_grid_neg_eta_avg_mod1] -> LVRT_detector/3(veta_n), frt_detection_inputs/3  "v_grid_neg_eta_avg"
  Step3/1 -> frt_detection_inputs/6, LVRT_detector/6(enable)  "enable"
  dvxi_p/dt/1(xdot_hat) -> Abs/1
  LVRT_detector/1(pwr_lim_enable) -> pwr_lim_enable/1  "pwr_lim_enable"
  dvxi_n/dt/1(xdot_hat) -> Abs1/1
  Step1/1 -> LVRT_detector/8(reset)
  red_dyn_enabled/1 -> LVRT_detector/7(red_dyn_enabled)
  LVRT_detector/2(frt_exceeded) -> frt_exceeded/1  "lvrt_exceeded"
  LVRT_detector/5(red_dyn_active) -> red_dyn_active/1
  LVRT_detector/4(frt_state) -> frt_state/1
  LVRT_detector/3(frt_active) -> frt_active/1
  Abs/1 -> frt_detection_inputs/4, LVRT_detector/4(vxi_p_dot)  "vxi_pos_dot"
  Abs1/1 -> frt_detection_inputs/5, LVRT_detector/5(vxi_n_dot)  "vxi_neg_dot"

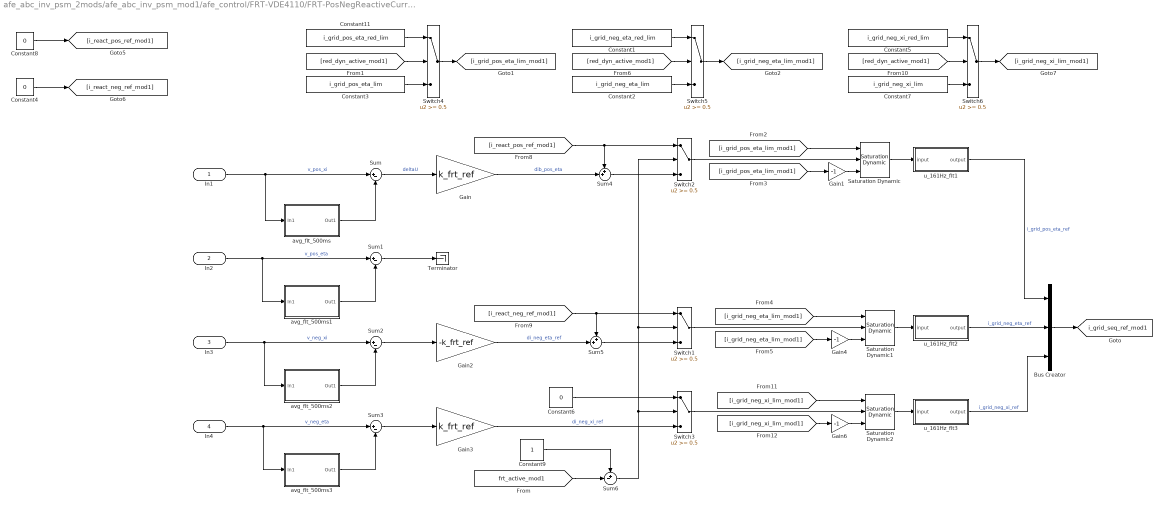
== system afe_abc_inv_psm_2mods/afe_abc_inv_psm_mod1/afe_control/FRT-VDE4110/FRT-PosNegReactiveCurrentReferences ==
  In1 : Inport
  In2 : Inport  Port=2
  In3 : Inport  Port=3
  In4 : Inport  Port=4
  Bus Creator : BusCreator  Inputs=3
  Constant1 : Constant  Value=i_grid_neg_eta_red_lim
  Constant11 : Constant  Value=i_grid_pos_eta_red_lim
  Constant2 : Constant  Value=i_grid_neg_eta_lim
  Constant3 : Constant  Value=i_grid_pos_eta_lim
  Constant4 : Constant  Value=0
  Constant5 : Constant  Value=i_grid_neg_xi_red_lim
  Constant6 : Constant  Value=0
  Constant7 : Constant  Value=i_grid_neg_xi_lim
  Constant8 : Constant  Value=0
  Constant9 : Constant
  Gain : Gain  Gain=k_frt_ref
  Gain1 : Gain  Gain=-1
  Gain2 : Gain  Gain=-k_frt_ref
  Gain3 : Gain  Gain=k_frt_ref
  Gain4 : Gain  Gain=-1
  Gain6 : Gain  Gain=-1
  Saturation Dynamic : simulink/Discontinuities/Saturation Dynamic  OutMin=[]  OutMax=[]  OutDataTypeStr=Inherit: Same as second input  OutDataType=fixdt(1, 16)  OutScaling=2^-10  DoSatur=off
  Saturation Dynamic1 : simulink/Discontinuities/Saturation Dynamic  OutMin=[]  OutMax=[]  OutDataTypeStr=Inherit: Same as second input  OutDataType=fixdt(1, 16)  OutScaling=2^-10  DoSatur=off
  Saturation Dynamic2 : simulink/Discontinuities/Saturation Dynamic  OutMin=[]  OutMax=[]  OutDataTypeStr=Inherit: Same as second input  OutDataType=fixdt(1, 16)  OutScaling=2^-10  DoSatur=off
  Sum{,1..3} (4 alike) : Sum  Inputs=|+-
  Sum4 : Sum  Inputs=++|
  Sum5 : Sum  Inputs=++|
  Sum6 : Sum  Inputs=+-|
  Switch{1..6} (6 alike) : Switch  Threshold=0.5  SaturateOnIntegerOverflow=off  InputSameDT=off
  Terminator : Terminator
  avg_flt_500ms : Subsystem
  avg_flt_500ms1 : Subsystem
  avg_flt_500ms2 : Subsystem
  avg_flt_500ms3 : Subsystem
  u_161Hz_flt1 : Subsystem
  u_161Hz_flt2 : Subsystem
  u_161Hz_flt3 : Subsystem
  tag scope: i_grid_seq_ref_mod1=global
  wires:
  In1/1 -> avg_flt_500ms/1(In1), Sum/1  "v_pos_xi"
  avg_flt_500ms/1(Out1) -> Sum/2
  Sum/1 -> Gain/1  "deltaU"
  Sum1/1 -> Terminator/1
  avg_flt_500ms1/1(Out1) -> Sum1/2
  In2/1 -> avg_flt_500ms1/1(In1), Sum1/1  "v_pos_eta"
  avg_flt_500ms3/1(Out1) -> Sum3/2
  Sum2/1 -> Gain2/1
  In3/1 -> avg_flt_500ms2/1(In1), Sum2/1  "v_neg_xi"
  avg_flt_500ms2/1(Out1) -> Sum2/2
  In4/1 -> avg_flt_500ms3/1(In1), Sum3/1  "v_neg_eta"
  Bus Creator/1 -> [i_grid_seq_ref_mod1]
  Gain/1 -> Sum4/2  "dib_pos_eta"
  [i_react_pos_ref_mod1] -> Switch2/1, Sum4/1
  Sum4/1 -> Switch2/3
  Switch2/1 -> Saturation Dynamic/2
  Saturation Dynamic/1 -> u_161Hz_flt1/1(input)
  Constant6/1 -> Switch3/1
  Gain3/1 -> Switch3/3  "di_neg_xi_ref"
  Sum6/1 -> Switch1/2, Switch2/2, Switch3/2
  Sum3/1 -> Gain3/1
  Gain2/1 -> Sum5/2  "di_neg_eta_ref"
  Sum5/1 -> Switch1/3
  [i_react_neg_ref_mod1] -> Switch1/1, Sum5/1
  Switch4/1 -> [i_grid_pos_eta_lim_mod1]
  [red_dyn_active_mod1] -> Switch4/2
  Constant3/1 -> Switch4/3
  Constant11/1 -> Switch4/1
  [i_grid_pos_eta_lim_mod1] -> Saturation Dynamic/1
  [i_grid_pos_eta_lim_mod1] -> Gain1/1
  Gain1/1 -> Saturation Dynamic/3
  Saturation Dynamic2/1 -> u_161Hz_flt3/1(input)
  Switch3/1 -> Saturation Dynamic2/2
  [i_grid_neg_xi_lim_mod1] -> Saturation Dynamic2/1
  [i_grid_neg_xi_lim_mod1] -> Gain6/1
  Gain4/1 -> Saturation Dynamic1/3
  [i_grid_neg_eta_lim_mod1] -> Gain4/1
  [i_grid_neg_eta_lim_mod1] -> Saturation Dynamic1/1
  Switch1/1 -> Saturation Dynamic1/2
  Saturation Dynamic1/1 -> u_161Hz_flt2/1(input)
  [red_dyn_active_mod1] -> Switch5/2
  Constant2/1 -> Switch5/3
  Constant1/1 -> Switch5/1
  Switch5/1 -> [i_grid_neg_eta_lim_mod1]
  Constant4/1 -> [i_react_neg_ref_mod1]
  Constant8/1 -> [i_react_pos_ref_mod1]
  Constant7/1 -> Switch6/3
  Switch6/1 -> [i_grid_neg_xi_lim_mod1]
  Constant5/1 -> Switch6/1
  [red_dyn_active_mod1] -> Switch6/2
  Gain6/1 -> Saturation Dynamic2/3
  u_161Hz_flt2/1(output) -> Bus Creator/2  "i_grid_neg_eta_ref"
  u_161Hz_flt3/1(output) -> Bus Creator/3  "i_grid_neg_xi_ref"
  u_161Hz_flt1/1(output) -> Bus Creator/1  "i_grid_pos_eta_ref"
  [frt_active_mod1] -> Sum6/2
  Constant9/1 -> Sum6/1

== system afe_abc_inv_psm_2mods/afe_abc_inv_psm_mod1/afe_control/current_ctrl/Inner Loop Current Control ==
  In1 : Inport
  is_abc : Inport  Port=2
  -1<x<1 : Saturate  UpperLimit=1  LowerLimit=-1
  Add : Sum
  Bus Creator1 : BusCreator  Inputs=2
  "Current-Control, Phase a" : Subsystem
  "Current-Control, Phase b" : Subsystem
  "Current-Control, Phase c" : Subsystem
  Demux1 : Demux  Outputs=3
  MATLAB Function : MATLAB Function  TreatAsAtomicUnit=on
  Mux : Mux  Inputs=3
  Selector : Selector  InputPortWidth=3  IndexOptions=Index vector (dialog)  Indices=[1]  OutputSizes=1
  Selector1 : Selector  InputPortWidth=3  IndexOptions=Index vector (dialog)  Indices=[1]  OutputSizes=1
  Selector2 : Selector  InputPortWidth=3  IndexOptions=Index vector (dialog)  Indices=[2]  OutputSizes=1
  Selector3 : Selector  InputPortWidth=3  IndexOptions=Index vector (dialog)  Indices=[2]  OutputSizes=1
  Selector4 : Selector  InputPortWidth=3  IndexOptions=Index vector (dialog)  Indices=[3]  OutputSizes=1
  Selector5 : Selector  InputPortWidth=3  IndexOptions=Index vector (dialog)  Indices=[3]  OutputSizes=1
  Unit Delay1 : UnitDelay  SampleTime=ts_afe  HasFrameUpgradeWarning=on
  Unit Delay2 : UnitDelay  SampleTime=ts_afe  HasFrameUpgradeWarning=on
  Unit Delay3 : UnitDelay  SampleTime=ts_afe  HasFrameUpgradeWarning=on
  afe_ictrl_out/afe_ictrl_ff : Scope  NumInputPorts=2
  isa_ref/isa : Scope  NumInputPorts=2
  isb_ref/isb : Scope  NumInputPorts=2
  isc_ref/isc : Scope  NumInputPorts=2
  uab : Outport  VectorParamsAs1DForOutWhenUnconnected=off
  wires:
  In1/1 -> Selector4/1, Selector2/1, Selector/1  "i_abc_ref"
  is_abc/1 -> Selector5/1, Selector3/1, Selector1/1  "i_abc"
  Add/1 -> -1<x<1/1  "v_abc"
  Selector/1 -> isa_ref/isa/1, "Current-Control, Phase a"/1(In1)  "isa_ref"
  Selector1/1 -> isa_ref/isa/2, "Current-Control, Phase a"/2(In2)  "isa"
  Selector2/1 -> isb_ref/isb/1, "Current-Control, Phase b"/1(In1)  "isb_ref"
  Selector3/1 -> isb_ref/isb/2, "Current-Control, Phase b"/2(In2)  "isb"
  Selector4/1 -> isc_ref/isc/1, "Current-Control, Phase c"/1(In1)  "isc_ref"
  Selector5/1 -> isc_ref/isc/2, "Current-Control, Phase c"/2(In2)  "isc"
  "Current-Control, Phase a"/1(Out1) -> Mux/1  "v_a"
  "Current-Control, Phase b"/1(Out1) -> Mux/2  "v_b"
  "Current-Control, Phase c"/1(Out1) -> Mux/3  "v_c"
  Mux/1 -> afe_ictrl_out/afe_ictrl_ff/1, Add/1  "v_abc"
  Demux1/3 -> MATLAB Function/3(c)  "v_c"
  MATLAB Function/1(alpha) -> Unit Delay2/1  "u_alpha"
  Unit Delay3/1 -> Bus Creator1/2  "ubeta_afe"
  Demux1/2 -> MATLAB Function/2(b)  "v_b"
  MATLAB Function/2(beta) -> Unit Delay3/1  "u_beta"
  Demux1/1 -> MATLAB Function/1(a)  "v_a"
  Unit Delay2/1 -> Bus Creator1/1  "ualpha_afe"
  Bus Creator1/1 -> uab/1
  -1<x<1/1 -> Demux1/1  "v_abc"
  Unit Delay1/1 -> afe_ictrl_out/afe_ictrl_ff/2
  [v_grid_ff_abc_mod1] -> Unit Delay1/1

== system afe_abc_inv_psm_2mods/afe_abc_inv_psm_mod1/afe_control/current_ctrl/current_transformation ==
  is_a_pu : Inport
  is_b_pu : Inport  Port=2
  is_c_pu : Inport  Port=3
  Bus Creator : BusCreator  Inputs=3
  alphabeta2xieta : MATLAB Function  TreatAsAtomicUnit=on  SystemSampleTime=ts_afe
  uvw2alphabeta : MATLAB Function  TreatAsAtomicUnit=on  SystemSampleTime=ts_afe
  tag scope: i_eta_pu_mod1=global, i_xi_pu_mod1=global, is_abc_pu_mod1=global
  wires:
  is_c_pu/1 -> Bus Creator/3, uvw2alphabeta/3(w)
  alphabeta2xieta/2(eta) -> [i_eta_pu_mod1]  "ieta_pu"
  alphabeta2xieta/1(xi) -> [i_xi_pu_mod1]  "ixi_pu"
  is_b_pu/1 -> Bus Creator/2, uvw2alphabeta/2(v)
  uvw2alphabeta/2(beta) -> alphabeta2xieta/2(beta)  "ibeta_pu"
  uvw2alphabeta/1(alpha) -> alphabeta2xieta/1(alpha)  "ialpha_pu"
  [gamma_grid_pll_mod1] -> alphabeta2xieta/3(gamma)
  is_a_pu/1 -> Bus Creator/1, uvw2alphabeta/1(u)
  Bus Creator/1 -> [is_abc_pu_mod1]

== system afe_abc_inv_psm_2mods/afe_abc_inv_psm_mod1/afe_control/current_ctrl/sample_hold_normalization ==
  is_a : Inport
  is_b : Inport  Port=2
  is_c : Inport  Port=3
  Gain : Gain  Gain=1/Igrid_phase_normalization_factor
  Gain1 : Gain  Gain=1/Igrid_phase_normalization_factor
  Gain2 : Gain  Gain=1/Igrid_phase_normalization_factor
  Quantizer : Quantizer  QuantizationInterval=adc_quantization
  Quantizer1 : Quantizer  QuantizationInterval=adc_quantization
  Quantizer2 : Quantizer  QuantizationInterval=adc_quantization
  Subsystem1 : Subsystem
      mask Display: disp('S/H afe mod 1');
  Subsystem2 : Subsystem
      mask Display: disp('S/H afe mod 1');
  Subsystem4 : Subsystem
      mask Display: disp('S/H afe mod 1');
  Unit Delay : UnitDelay  SampleTime=ts_afe  HasFrameUpgradeWarning=on
  Unit Delay1 : UnitDelay  SampleTime=ts_afe  HasFrameUpgradeWarning=on
  Unit Delay2 : UnitDelay  SampleTime=ts_afe  HasFrameUpgradeWarning=on
  is_a_pu : Outport
  is_b_pu : Outport  Port=2
  is_c_pu : Outport  Port=3
  wires:
  is_a/1 -> Gain/1
  Quantizer/1 -> Subsystem1/1(In)
  is_c/1 -> Gain2/1
  is_b/1 -> Gain1/1
  Unit Delay/1 -> is_a_pu/1
  Unit Delay1/1 -> is_b_pu/1
  Unit Delay2/1 -> is_c_pu/1
  Quantizer1/1 -> Subsystem2/1(In)
  Quantizer2/1 -> Subsystem4/1(In)
  Subsystem1/1(Out) -> Unit Delay/1
  Subsystem2/1(Out) -> Unit Delay1/1
  Subsystem4/1(Out) -> Unit Delay2/1
  Gain/1 -> Quantizer/1
  Gain1/1 -> Quantizer1/1
  Gain2/1 -> Quantizer2/1

== system afe_abc_inv_psm_2mods/afe_abc_inv_psm_mod1/afe_control/current_ctrl/xieta2abc ==
  pos_xi : Inport
  pos_eta : Inport  Port=2
  neg_xi : Inport  Port=3
  neg_eta : Inport  Port=4
  gamma : Inport  Port=5
  MATLAB Function2 : MATLAB Function  TreatAsAtomicUnit=on  SystemSampleTime=ts_afe
  Mux : Mux  Inputs=3
  Negative Sequence : MATLAB Function  TreatAsAtomicUnit=on  SystemSampleTime=ts_afe
  Positive Sequence : MATLAB Function  TreatAsAtomicUnit=on  SystemSampleTime=ts_afe
  Sum : Sum  Inputs=|++
  Sum1 : Sum  Inputs=|++
  i_abc : Outport
  wires:
  neg_eta/1 -> Negative Sequence/2(eta)
  MATLAB Function2/1(a) -> Mux/1  "i_a"
  Positive Sequence/2(beta) -> Sum1/1
  Sum/1 -> MATLAB Function2/1(alpha)
  gamma/1 -> Negative Sequence/3(gamma), Positive Sequence/3(gamma)
  MATLAB Function2/3(c) -> Mux/3  "i_c"
  Negative Sequence/1(alpha) -> Sum/2
  Positive Sequence/1(alpha) -> Sum/1
  Negative Sequence/2(beta) -> Sum1/2
  MATLAB Function2/2(b) -> Mux/2  "i_b"
  Sum1/1 -> MATLAB Function2/2(beta)
  neg_xi/1 -> Negative Sequence/1(xi)
  pos_xi/1 -> Positive Sequence/1(xi)
  pos_eta/1 -> Positive Sequence/2(eta)
  Mux/1 -> i_abc/1  "i_abc"

== system afe_abc_inv_psm_2mods/afe_abc_inv_psm_mod1/afe_control/current_sequence_avg/average_filter_ccaller ==
  i_grid_pos_xi : Inport
  i_grid_pos_eta : Inport  Port=2
  i_grid_neg_xi : Inport  Port=3
  i_grid_neg_eta : Inport  Port=4
  Moving Average Filter5 : Subsystem
  Moving Average Filter6 : Subsystem
  Moving Average Filter7 : Subsystem
  Moving Average Filter8 : Subsystem
  i_grid_pos_xi_avg : Outport
  i_grid_pos_eta_avg : Outport  Port=2
  i_grid_neg_xi_avg : Outport  Port=3
  i_grid_neg_eta_avg : Outport  Port=4
  wires:
  Moving Average Filter6/1(xi) -> i_grid_pos_eta_avg/1
  [omega_grid_pll_mod1] -> Moving Average Filter5/2(In3), Moving Average Filter8/2(In3), Moving Average Filter7/2(In3), Moving Average Filter6/2(In3)
  i_grid_pos_eta/1 -> Moving Average Filter6/1(In2)
  Moving Average Filter8/1(xi) -> i_grid_neg_eta_avg/1
  i_grid_neg_xi/1 -> Moving Average Filter7/1(In2)
  Moving Average Filter7/1(xi) -> i_grid_neg_xi_avg/1
  i_grid_pos_xi/1 -> Moving Average Filter5/1(In2)
  i_grid_neg_eta/1 -> Moving Average Filter8/1(In2)
  Moving Average Filter5/1(xi) -> i_grid_pos_xi_avg/1

== system afe_abc_inv_psm_2mods/afe_abc_inv_psm_mod1/afe_control/current_sequence_avg/average_filter_simulink ==
  i_grid_pos_xi : Inport
  i_grid_pos_eta : Inport  Port=2
  i_grid_neg_xi : Inport  Port=3
  i_grid_neg_eta : Inport  Port=4
  moving_avarage1 : Subsystem
  moving_avarage2 : Subsystem
  moving_avarage3 : Subsystem
  moving_avarage4 : Subsystem
  i_grid_pos_xi_avg : Outport
  i_grid_pos_eta_avg : Outport  Port=2
  i_grid_neg_xi_avg : Outport  Port=3
  i_grid_neg_eta_avg : Outport  Port=4
  wires:
  moving_avarage3/1(Mean) -> i_grid_neg_xi_avg/1
  moving_avarage1/1(Mean) -> i_grid_pos_xi_avg/1
  i_grid_pos_eta/1 -> moving_avarage2/1(In)
  i_grid_neg_eta/1 -> moving_avarage4/1(In)
  i_grid_pos_xi/1 -> moving_avarage1/1(In)
  moving_avarage4/1(Mean) -> i_grid_neg_eta_avg/1
  i_grid_neg_xi/1 -> moving_avarage3/1(In)
  moving_avarage2/1(Mean) -> i_grid_pos_eta_avg/1

== system afe_abc_inv_psm_2mods/afe_abc_inv_psm_mod1/afe_control/grid_current_sampling_and_alpha_beta_transformation/sample_hold_normalization ==
  ig_a : Inport
  ig_b : Inport  Port=2
  ig_c : Inport  Port=3
  Gain1 : Gain  Gain=1/Igrid_phase_normalization_factor
  Gain2 : Gain  Gain=1/Igrid_phase_normalization_factor
  Gain3 : Gain  Gain=1/Igrid_phase_normalization_factor
  Gain4 : Gain  Gain=-1
  Gain5 : Gain  Gain=-1
  Gain6 : Gain  Gain=-1
  Quantizer1 : Quantizer  QuantizationInterval=adc_quantization
  Quantizer2 : Quantizer  QuantizationInterval=adc_quantization
  Quantizer4 : Quantizer  QuantizationInterval=adc_quantization
  Subsystem1 : Subsystem
      mask Display: disp('S/H afe mod 1');
  Subsystem2 : Subsystem
      mask Display: disp('S/H afe mod 1');
  Subsystem3 : Subsystem
      mask Display: disp('S/H afe mod 1');
  Unit Delay : UnitDelay  SampleTime=ts_afe  HasFrameUpgradeWarning=on
  Unit Delay1 : UnitDelay  SampleTime=ts_afe  HasFrameUpgradeWarning=on
  Unit Delay2 : UnitDelay  SampleTime=ts_afe  HasFrameUpgradeWarning=on
  ig_a_pu : Outport
  ig_b_pu : Outport  Port=2
  ig_c_pu : Outport  Port=3
  wires:
  Subsystem2/1(Out) -> Unit Delay1/1
  Subsystem1/1(Out) -> Unit Delay/1
  Subsystem3/1(Out) -> Unit Delay2/1
  Quantizer4/1 -> Subsystem1/1(In)
  Quantizer1/1 -> Subsystem2/1(In)
  Quantizer2/1 -> Subsystem3/1(In)
  Gain3/1 -> Quantizer4/1
  Gain1/1 -> Quantizer1/1
  Gain2/1 -> Quantizer2/1
  ig_a/1 -> Gain3/1
  ig_b/1 -> Gain1/1
  ig_c/1 -> Gain2/1
  Unit Delay/1 -> Gain4/1
  Unit Delay1/1 -> Gain5/1
  Unit Delay2/1 -> Gain6/1
  Gain4/1 -> ig_a_pu/1
  Gain5/1 -> ig_b_pu/1
  Gain6/1 -> ig_c_pu/1

== system afe_abc_inv_psm_2mods/afe_abc_inv_psm_mod1/afe_control/grid_voltage_phase_lock_loops/DDSRF-PLL ==
  pll_stageA : Subsystem
  pll_stageB : Subsystem
  grid_phase_out : Outport
  wires:
  pll_stageB/1(wt_grid) -> pll_stageA/1(gamma_grid), grid_phase_out/1
  pll_stageA/2(u_grid_pos_eta) -> pll_stageB/2(u_grid_pos_eta)  "u_grid_pos_eta"
  pll_stageA/1(u_grid_pos_xi) -> pll_stageB/1(u_grid_pos_xi)  "u_grid_pos_xi"

== system afe_abc_inv_psm_2mods/afe_abc_inv_psm_mod1/afe_control/grid_voltage_phase_lock_loops/DQ-PLL ==
  pll_stageA : Subsystem
  pll_stageB : Subsystem
  grid_phase_out : Outport
  wires:
  pll_stageA/2(u_grid_pos_eta) -> pll_stageB/2(u_grid_pos_eta)  "u_grid_pos_eta"
  pll_stageB/1(gamma_grid_pll) -> pll_stageA/1(gamma_grid), grid_phase_out/1
  pll_stageA/1(u_grid_pos_xi) -> pll_stageB/1(u_grid_pos_xi)  "u_grid_pos_xi"
